simulink model "M1_P2_D"  (R2023a)
settings: Solver=VariableStepAuto  StartTime=0.0  StopTime=3  RelTol=1e-3
undefined symbols (not defined in the file): f_eff, J_eff, Kb, Ktn, L, R
settings Model: Creator=azzam  LastModifiedBy=azzam

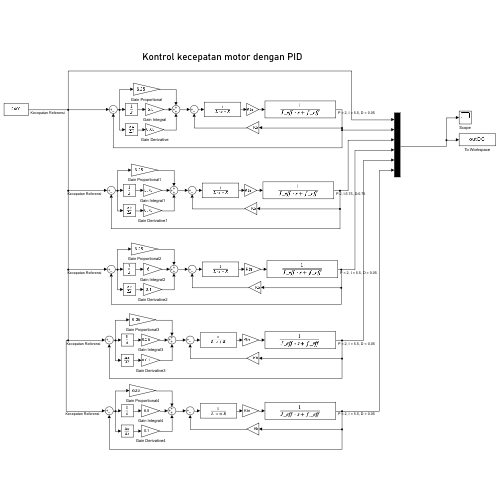
[thumbnail: Simulink's stored preview of the top-level diagram]
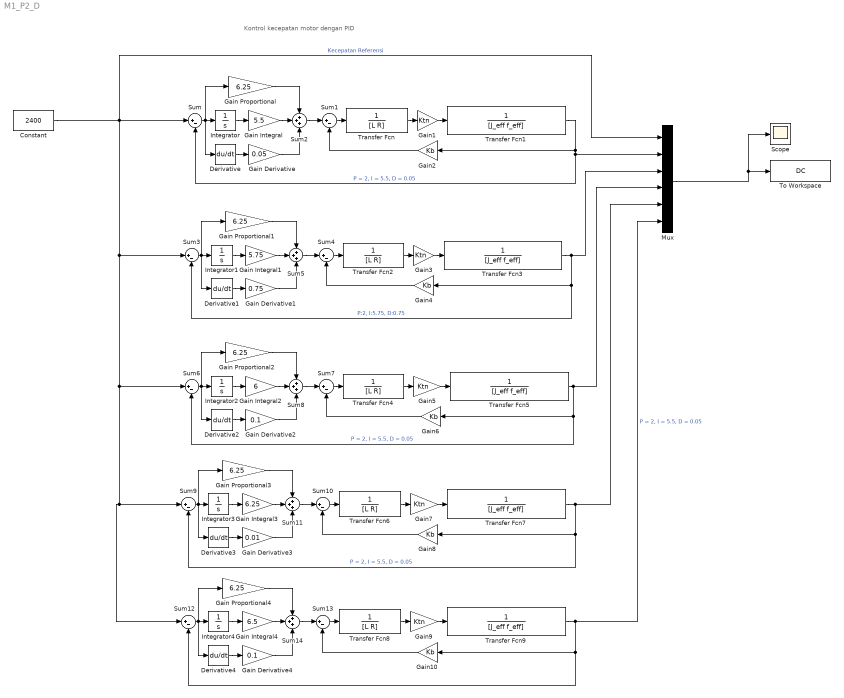
== system M1_P2_D ==
  note: Kontrol kecepatan motor dengan PID
  Constant : Constant  Value=2400
  Derivative{,1..4} (5 alike) : Derivative
  Gain Derivative : Gain  Gain=0.05
  Gain Derivative1 : Gain  Gain=0.75
  Gain Derivative2 : Gain  Gain=0.1
  Gain Derivative3 : Gain  Gain=0.01
  Gain Derivative4 : Gain  Gain=0.1
  Gain Integral : Gain  Gain=5.5
  Gain Integral1 : Gain  Gain=5.75
  Gain Integral2 : Gain  Gain=6
  Gain Integral3 : Gain  Gain=6.25
  Gain Integral4 : Gain  Gain=6.5
  Gain Proportional{,1..4} (5 alike) : Gain  Gain=6.25
  Gain{1,3,5,7,9} (5 alike) : Gain  Gain=Ktn
  Gain{2,4,6,8,10} (5 alike) : Gain  Gain=Kb
  Integrator{,1..4} (5 alike) : Integrator
  Mux : Mux  Inputs=6
  Scope : Scope
  Sum{,1,3..4,6..7,9..10,12..13} (10 alike) : Sum  Inputs=|+-
  Sum{2,5,8,11,14} (5 alike) : Sum  Inputs=+++
  To Workspace : ToWorkspace  VariableName=DC  SaveFormat=Timeseries  SampleTime=-1
  Transfer Fcn{,2,4,6,8} (5 alike) : TransferFcn  Denominator=[L R]
  Transfer Fcn{1,3,5,7,9} (5 alike) : TransferFcn  Denominator=[J_eff f_eff]
  wires:
  Mux/1 -> To Workspace/1, Scope/1
  Gain1/1 -> Transfer Fcn1/1
  Sum1/1 -> Transfer Fcn/1
  Gain Proportional/1 -> Sum2/1
  Derivative/1 -> Gain Derivative/1
  Transfer Fcn1/1 -> Sum/2, Mux/2, Gain2/1  "P = 2, I = 5.5, D = 0.05"
  Gain2/1 -> Sum1/2
  Sum2/1 -> Sum1/1
  Transfer Fcn/1 -> Gain1/1
  Sum/1 -> Integrator/1, Derivative/1, Gain Proportional/1
  Gain Derivative/1 -> Sum2/3
  Gain Integral/1 -> Sum2/2
  Integrator/1 -> Gain Integral/1
  Integrator1/1 -> Gain Integral1/1
  Gain Integral1/1 -> Sum5/2
  Gain Derivative1/1 -> Sum5/3
  Sum3/1 -> Integrator1/1, Derivative1/1, Gain Proportional1/1
  Transfer Fcn2/1 -> Gain3/1
  Sum5/1 -> Sum4/1
  Gain4/1 -> Sum4/2
  Transfer Fcn3/1 -> Sum3/2, Gain4/1, Mux/3  "P:2, I:5.75, D:0.75"
  Derivative1/1 -> Gain Derivative1/1
  Sum4/1 -> Transfer Fcn2/1
  Gain3/1 -> Transfer Fcn3/1
  Gain Proportional1/1 -> Sum5/1
  Gain Proportional2/1 -> Sum8/1
  Sum7/1 -> Transfer Fcn4/1
  Derivative2/1 -> Gain Derivative2/1
  Transfer Fcn5/1 -> Sum6/2, Gain6/1, Mux/4  "P = 2, I = 5.5, D = 0.05"
  Gain Integral2/1 -> Sum8/2
  Gain Derivative2/1 -> Sum8/3
  Sum6/1 -> Integrator2/1, Derivative2/1, Gain Proportional2/1
  Transfer Fcn4/1 -> Gain5/1
  Sum8/1 -> Sum7/1
  Gain5/1 -> Transfer Fcn5/1
  Integrator2/1 -> Gain Integral2/1
  Gain6/1 -> Sum7/2
  Gain Proportional3/1 -> Sum11/1
  Transfer Fcn7/1 -> Mux/5, Sum9/2, Gain8/1  "P = 2, I = 5.5, D = 0.05"
  Gain8/1 -> Sum10/2
  Sum10/1 -> Transfer Fcn6/1
  Transfer Fcn6/1 -> Gain7/1
  Integrator3/1 -> Gain Integral3/1
  Sum9/1 -> Integrator3/1, Derivative3/1, Gain Proportional3/1
  Derivative3/1 -> Gain Derivative3/1
  Gain Integral3/1 -> Sum11/2
  Sum11/1 -> Sum10/1
  Gain Derivative3/1 -> Sum11/3
  Gain7/1 -> Transfer Fcn7/1
  Constant/1 -> Sum12/1, Sum9/1, Sum6/1, Sum3/1, Mux/1, Sum/1  "Kecepatan Referensi"
  Gain Proportional4/1 -> Sum14/1
  Transfer Fcn9/1 -> Mux/6, Sum12/2, Gain10/1  "P = 2, I = 5.5, D = 0.05"
  Gain10/1 -> Sum13/2
  Sum13/1 -> Transfer Fcn8/1
  Transfer Fcn8/1 -> Gain9/1
  Integrator4/1 -> Gain Integral4/1
  Sum12/1 -> Integrator4/1, Derivative4/1, Gain Proportional4/1
  Derivative4/1 -> Gain Derivative4/1
  Gain Integral4/1 -> Sum14/2
  Sum14/1 -> Sum13/1
  Gain Derivative4/1 -> Sum14/3
  Gain9/1 -> Transfer Fcn9/1
